simulink model "Tra_Prt"  (R2016b)
settings: configuration reference "CodeGenConfigSet" (kept outside this file)
values from neighbouring files (symbols this model uses):
  Tra_dtrqPTORmpP_Neg_C = Calibration.Parameter    [init_Tra_Prt.m]
  Tra_dtrqPTORmpP_Pos_C = Calibration.Parameter    [init_Tra_Prt.m]
  Tra_numGearGrpThres1_C = Calibration.Parameter    [init_Tra_Prt.m]
  Tra_numGearGrpThres2_C = Calibration.Parameter    [init_Tra_Prt.m]
  Tra_numGearGrpThres3_C = Calibration.Parameter    [init_Tra_Prt.m]
  Tra_numGearGrpThres4_C = Calibration.Parameter    [init_Tra_Prt.m]
  Tra_numGearGrpThres5_C = Calibration.Parameter    [init_Tra_Prt.m]
  Tra_swtPTOLim1KD_C = Calibration.Parameter    [init_Tra_Prt.m]
  Tra_trqInMax_C = Calibration.Parameter    [init_Tra_Prt.m]
  Tra_trqMaxGearGrp1_CUR = Calibration.Parameter    [init_Tra_Prt.m]
  Tra_trqMaxGearGrp1_CURX = Calibration.Parameter    [init_Tra_Prt.m]
  Tra_trqMaxGearGrp2_CUR = Calibration.Parameter    [init_Tra_Prt.m]
  Tra_trqMaxGearGrp2_CURX = Calibration.Parameter    [init_Tra_Prt.m]
  Tra_trqMaxGearGrp3_CUR = Calibration.Parameter    [init_Tra_Prt.m]
  Tra_trqMaxGearGrp3_CURX = Calibration.Parameter    [init_Tra_Prt.m]
  Tra_trqMaxGearGrp4_CUR = Calibration.Parameter    [init_Tra_Prt.m]
  Tra_trqMaxGearGrp4_CURX = Calibration.Parameter    [init_Tra_Prt.m]
  Tra_trqMaxGearGrp5_CUR = Calibration.Parameter    [init_Tra_Prt.m]
  Tra_trqMaxGearGrp5_CURX = Calibration.Parameter    [init_Tra_Prt.m]
  Tra_trqMaxGearGrp6_CUR = Calibration.Parameter    [init_Tra_Prt.m]
  Tra_trqMaxGearGrp6_CURX = Calibration.Parameter    [init_Tra_Prt.m]
  Tra_trqPTOLim1_CUR = Calibration.Parameter    [init_Tra_Prt.m]
  Tra_trqPTOLim1_CURX = Calibration.Parameter    [init_Tra_Prt.m]
  Tra_trqPTOLim2_CUR = Calibration.Parameter    [init_Tra_Prt.m]
  Tra_trqPTOLim2_CURX = Calibration.Parameter    [init_Tra_Prt.m]
  Tra_trqPTOLim3_CUR = Calibration.Parameter    [init_Tra_Prt.m]
  Tra_trqPTOLim3_CURX = Calibration.Parameter    [init_Tra_Prt.m]
  Tra_trqWESDemLim0_C = Calibration.Parameter    [init_Tra_Prt.m]
  Tra_trqWESDemLim1_C = Calibration.Parameter    [init_Tra_Prt.m]
  Tra_trqWESDemLim2_C = Calibration.Parameter    [init_Tra_Prt.m]
  Tra_trqWESDemLim3_C = Calibration.Parameter    [init_Tra_Prt.m]
undefined symbols (not defined in the file or in its folder): CEngDsT_tTransf_CURX, WESDem_State_conv
libraries: CXLib x1
settings Model: Creator=Colin  LastModifiedBy=wangrui
settings ConfigSetRef: SourceLocation=Base Workspace

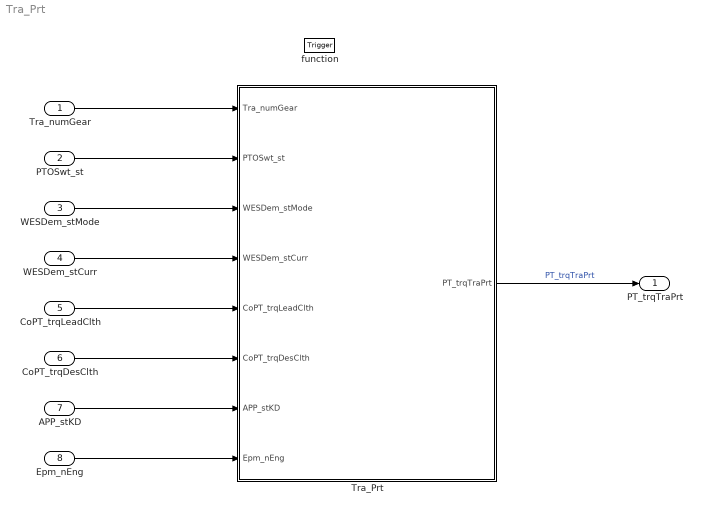
== system Tra_Prt ==
  Tra_numGear : Inport  Description=Current gear information  OutMin=-128  OutMax=127  OutDataTypeStr=Tra_num
  PTOSwt_st : Inport  Description=Power Take-off switch current state for a specific input voltage  Port=2  OutMin=0  OutMax=255  OutDataTypeStr=State_uint8
  WESDem_stMode : Inport  Description=Operating mode of the working engine speed demand  Port=3  OutMin=0  OutMax=255  OutDataTypeStr=State_uint8
  WESDem_stCurr : Inport  Description=Status of the working engine Speed Control  Port=4  OutDataTypeStr=Enum: WESDem_State_conv
  CoPT_trqLeadClth : Inport  Tag=Nm  Description=Lead torque demand at gearbox  Port=5  OutMin=-3000  OutMax=3000  OutDataTypeStr=Trq_Nm
  CoPT_trqDesClth : Inport  Tag=Nm  Description=Desired Clutch Torque  Port=6  OutMin=-3000  OutMax=3000  OutDataTypeStr=Trq_Nm
  APP_stKD : Inport  Description=State of accelerator pedal kick down  Port=7  OutMin=0  OutMax=1  OutDataTypeStr=boolean
  Epm_nEng : Inport  Tag=rpm  Description=Engine speed  Port=8  OutMin=0  OutMax=6000  OutDataTypeStr=EngSpeed_rpm
  function : TriggerPort  TriggerType=function-call  VariantControl=Variant
  Tra_Prt : Subsystem  RTWFcnName=Tra_Prt_Co  RTWFileName=Tra_Prt
      settings: RTWSystemCode=Nonreusable function  RTWFcnNameOpts=User specified  RTWFileNameOpts=User specified
  PT_trqTraPrt : Outport  Tag=Nm  Description=Maximum allowed inner torque  OutMin=-3000  OutMax=3000  OutDataTypeStr=Trq_Nm
  wires:
  Tra_Prt/1(PT_trqTraPrt) -> PT_trqTraPrt/1  "PT_trqTraPrt"
  Tra_numGear/1 -> Tra_Prt/1(Tra_numGear)
  PTOSwt_st/1 -> Tra_Prt/2(PTOSwt_st)
  WESDem_stMode/1 -> Tra_Prt/3(WESDem_stMode)
  WESDem_stCurr/1 -> Tra_Prt/4(WESDem_stCurr)
  CoPT_trqLeadClth/1 -> Tra_Prt/5(CoPT_trqLeadClth)
  APP_stKD/1 -> Tra_Prt/7(APP_stKD)
  CoPT_trqDesClth/1 -> Tra_Prt/6(CoPT_trqDesClth)
  Epm_nEng/1 -> Tra_Prt/8(Epm_nEng)

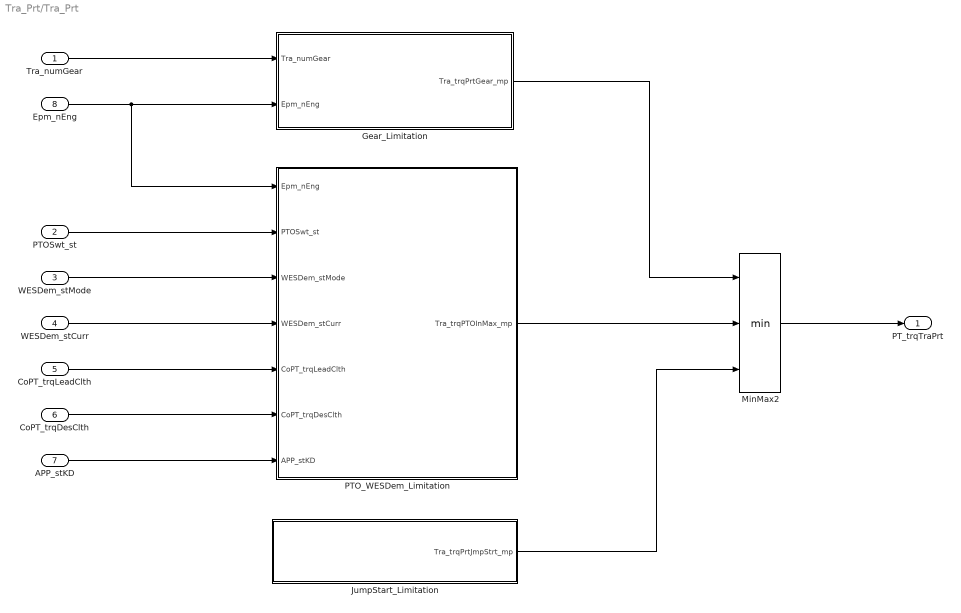
== system Tra_Prt/Tra_Prt ==
  Tra_numGear : Inport
  PTOSwt_st : Inport  Port=2
  WESDem_stMode : Inport  Port=3
  WESDem_stCurr : Inport  Port=4
  CoPT_trqLeadClth : Inport  Port=5
  CoPT_trqDesClth : Inport  Port=6
  APP_stKD : Inport  Port=7
  Epm_nEng : Inport  Port=8
  Gear_Limitation : Subsystem
  JumpStart_Limitation : Subsystem
  MinMax2 : MinMax  Inputs=3  InputSameDT=on
  PTO_WESDem_Limitation : Subsystem
  PT_trqTraPrt : Outport
  wires:
  Tra_numGear/1 -> Gear_Limitation/1(Tra_numGear)
  Gear_Limitation/1(Tra_trqPrtGear_mp) -> MinMax2/1
  MinMax2/1 -> PT_trqTraPrt/1
  APP_stKD/1 -> PTO_WESDem_Limitation/7(APP_stKD)
  CoPT_trqDesClth/1 -> PTO_WESDem_Limitation/6(CoPT_trqDesClth)
  PTO_WESDem_Limitation/1(Tra_trqPTOInMax_mp) -> MinMax2/2
  PTOSwt_st/1 -> PTO_WESDem_Limitation/2(PTOSwt_st)
  WESDem_stCurr/1 -> PTO_WESDem_Limitation/4(WESDem_stCurr)
  WESDem_stMode/1 -> PTO_WESDem_Limitation/3(WESDem_stMode)
  CoPT_trqLeadClth/1 -> PTO_WESDem_Limitation/5(CoPT_trqLeadClth)
  JumpStart_Limitation/1(Tra_trqPrtJmpStrt_mp) -> MinMax2/3
  Epm_nEng/1 -> PTO_WESDem_Limitation/1(Epm_nEng), Gear_Limitation/2(Epm_nEng)

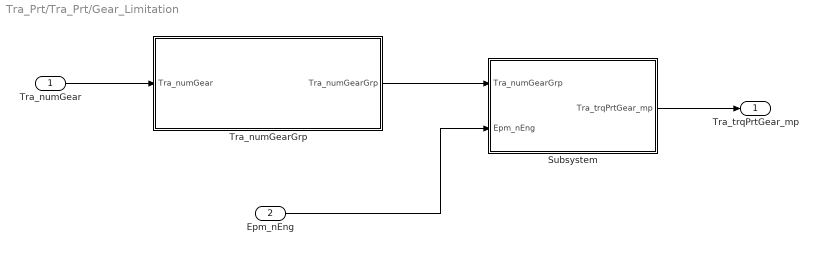
== system Tra_Prt/Tra_Prt/Gear_Limitation ==
  Tra_numGear : Inport
  Epm_nEng : Inport  Port=2
  Subsystem : Subsystem
  Tra_numGearGrp : Subsystem
  Tra_trqPrtGear_mp : Outport
  wires:
  Tra_numGear/1 -> Tra_numGearGrp/1(Tra_numGear)
  Tra_numGearGrp/1(Tra_numGearGrp) -> Subsystem/1(Tra_numGearGrp)
  Epm_nEng/1 -> Subsystem/2(Epm_nEng)
  Subsystem/1(Tra_trqPrtGear_mp) -> Tra_trqPrtGear_mp/1

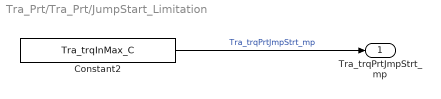
== system Tra_Prt/Tra_Prt/JumpStart_Limitation ==
  Constant2 : Constant  RequirementInfo={} %GIDa_d51cce05_4451_4a37_be15_ce81718d51d3  Value=Tra_trqInMax_C
  Tra_trqPrtJmpStrt_mp : Outport
  wires:
  Constant2/1 -> Tra_trqPrtJmpStrt_mp/1  "Tra_trqPrtJmpStrt_mp"

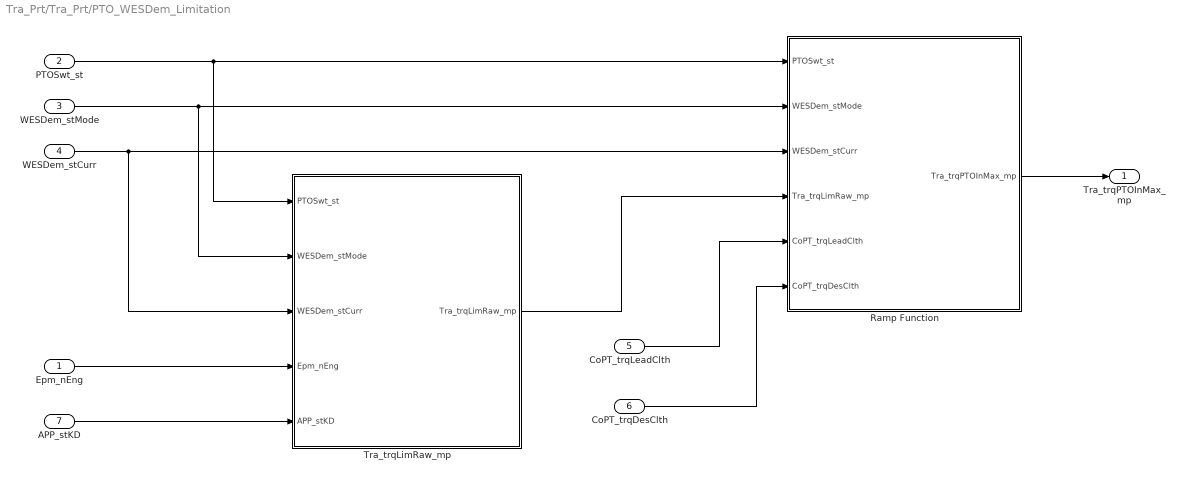
== system Tra_Prt/Tra_Prt/PTO_WESDem_Limitation ==
  Epm_nEng : Inport
  PTOSwt_st : Inport  Port=2
  WESDem_stMode : Inport  Port=3
  WESDem_stCurr : Inport  Port=4
  CoPT_trqLeadClth : Inport  Port=5
  CoPT_trqDesClth : Inport  Port=6
  APP_stKD : Inport  Port=7
  Ramp Function : Subsystem
  Tra_trqLimRaw_mp : Subsystem
  Tra_trqPTOInMax_mp : Outport
  wires:
  PTOSwt_st/1 -> Tra_trqLimRaw_mp/1(PTOSwt_st), Ramp Function/1(PTOSwt_st)
  WESDem_stMode/1 -> Tra_trqLimRaw_mp/2(WESDem_stMode), Ramp Function/2(WESDem_stMode)
  WESDem_stCurr/1 -> Tra_trqLimRaw_mp/3(WESDem_stCurr), Ramp Function/3(WESDem_stCurr)
  Ramp Function/1(Tra_trqPTOInMax_mp) -> Tra_trqPTOInMax_mp/1
  CoPT_trqLeadClth/1 -> Ramp Function/5(CoPT_trqLeadClth)
  CoPT_trqDesClth/1 -> Ramp Function/6(CoPT_trqDesClth)
  Epm_nEng/1 -> Tra_trqLimRaw_mp/4(Epm_nEng)
  APP_stKD/1 -> Tra_trqLimRaw_mp/5(APP_stKD)
  Tra_trqLimRaw_mp/1(Tra_trqLimRaw_mp) -> Ramp Function/4(Tra_trqLimRaw_mp)

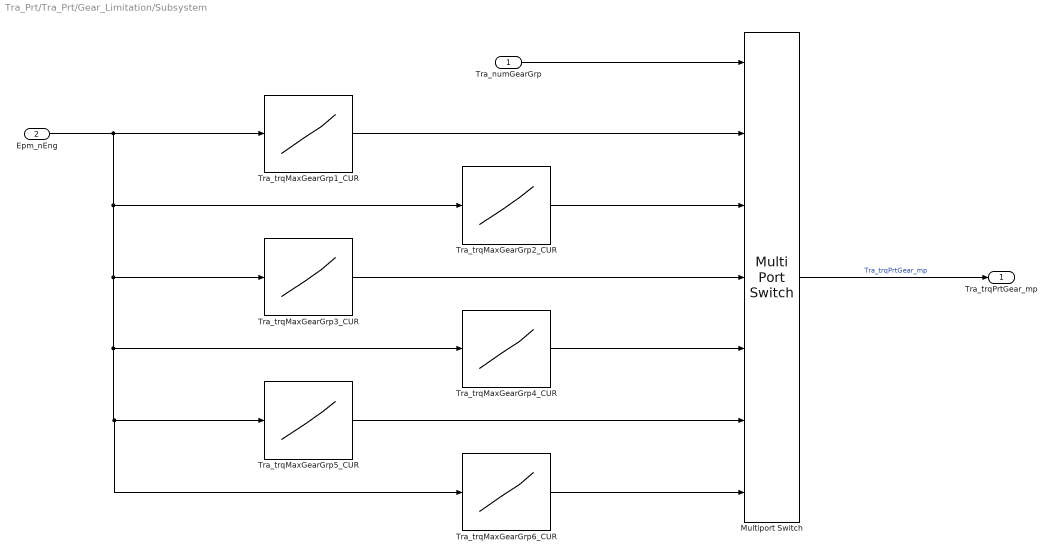
== system Tra_Prt/Tra_Prt/Gear_Limitation/Subsystem ==
  Tra_numGearGrp : Inport
  Epm_nEng : Inport  Port=2
  Multiport Switch : MultiPortSwitch  Inputs=6  InputSameDT=on
  Tra_trqMaxGearGrp1_CUR : Lookup_n-D  RequirementInfo={} %GIDa_9bf8303a_3058_4db5_a525_07331b8eeae7  DialogController=Simulink.DDGSource  NumberOfTableDimensions=1  BreakpointsForDimension1=Tra_trqMaxGearGrp1_CURX  BreakpointsForDimension2=CEngDsT_tTransf_CURX  IndexSearchMethod=Linear search  BeginIndexSearchUsingPreviousIndexResult=on  Table=Tra_trqMaxGearGrp1_CUR  ExtrapMethod=Clip  UseLastTableValue=on  InternalRulePriority=Speed  OutDataTypeStr=Inherit: Inherit via back propagation  SaturateOnIntegerOverflow=on
  Tra_trqMaxGearGrp2_CUR : Lookup_n-D  RequirementInfo={} %GIDa_3f32d6d9_4cb8_4f48_9c57_2c19b3164e61  DialogController=Simulink.DDGSource  NumberOfTableDimensions=1  BreakpointsForDimension1=Tra_trqMaxGearGrp2_CURX  BreakpointsForDimension2=CEngDsT_tTransf_CURX  IndexSearchMethod=Linear search  BeginIndexSearchUsingPreviousIndexResult=on  Table=Tra_trqMaxGearGrp2_CUR  ExtrapMethod=Clip  UseLastTableValue=on  InternalRulePriority=Speed  OutDataTypeStr=Inherit: Inherit via back propagation  SaturateOnIntegerOverflow=on
  Tra_trqMaxGearGrp3_CUR : Lookup_n-D  RequirementInfo={} %GIDa_1f71405c_5e82_4c6f_b5e1_f98a14c9db68  DialogController=Simulink.DDGSource  NumberOfTableDimensions=1  BreakpointsForDimension1=Tra_trqMaxGearGrp3_CURX  BreakpointsForDimension2=CEngDsT_tTransf_CURX  IndexSearchMethod=Linear search  BeginIndexSearchUsingPreviousIndexResult=on  Table=Tra_trqMaxGearGrp3_CUR  ExtrapMethod=Clip  UseLastTableValue=on  InternalRulePriority=Speed  OutDataTypeStr=Inherit: Inherit via back propagation  SaturateOnIntegerOverflow=on
  Tra_trqMaxGearGrp4_CUR : Lookup_n-D  RequirementInfo={} %GIDa_d67459b0_9d68_4b26_8ae3_ca0e9adf24a9  DialogController=Simulink.DDGSource  NumberOfTableDimensions=1  BreakpointsForDimension1=Tra_trqMaxGearGrp4_CURX  BreakpointsForDimension2=CEngDsT_tTransf_CURX  IndexSearchMethod=Linear search  BeginIndexSearchUsingPreviousIndexResult=on  Table=Tra_trqMaxGearGrp4_CUR  ExtrapMethod=Clip  UseLastTableValue=on  InternalRulePriority=Speed  OutDataTypeStr=Inherit: Inherit via back propagation  SaturateOnIntegerOverflow=on
  Tra_trqMaxGearGrp5_CUR : Lookup_n-D  RequirementInfo={} %GIDa_4c84db78_f469_4b3e_ba9a_5984f4299043  DialogController=Simulink.DDGSource  NumberOfTableDimensions=1  BreakpointsForDimension1=Tra_trqMaxGearGrp5_CURX  BreakpointsForDimension2=CEngDsT_tTransf_CURX  IndexSearchMethod=Linear search  BeginIndexSearchUsingPreviousIndexResult=on  Table=Tra_trqMaxGearGrp5_CUR  ExtrapMethod=Clip  UseLastTableValue=on  InternalRulePriority=Speed  OutDataTypeStr=Inherit: Inherit via back propagation  SaturateOnIntegerOverflow=on
  Tra_trqMaxGearGrp6_CUR : Lookup_n-D  RequirementInfo={} %GIDa_1b105f65_424f_42a0_97b6_462d21eb7e5b  DialogController=Simulink.DDGSource  NumberOfTableDimensions=1  BreakpointsForDimension1=Tra_trqMaxGearGrp6_CURX  BreakpointsForDimension2=CEngDsT_tTransf_CURX  IndexSearchMethod=Linear search  BeginIndexSearchUsingPreviousIndexResult=on  Table=Tra_trqMaxGearGrp6_CUR  ExtrapMethod=Clip  UseLastTableValue=on  InternalRulePriority=Speed  OutDataTypeStr=Inherit: Inherit via back propagation  SaturateOnIntegerOverflow=on
  Tra_trqPrtGear_mp : Outport
  wires:
  Tra_numGearGrp/1 -> Multiport Switch/1
  Multiport Switch/1 -> Tra_trqPrtGear_mp/1  "Tra_trqPrtGear_mp"
  Tra_trqMaxGearGrp3_CUR/1 -> Multiport Switch/4
  Tra_trqMaxGearGrp4_CUR/1 -> Multiport Switch/5
  Epm_nEng/1 -> Tra_trqMaxGearGrp1_CUR/1, Tra_trqMaxGearGrp2_CUR/1, Tra_trqMaxGearGrp5_CUR/1, Tra_trqMaxGearGrp6_CUR/1, Tra_trqMaxGearGrp4_CUR/1, Tra_trqMaxGearGrp3_CUR/1
  Tra_trqMaxGearGrp6_CUR/1 -> Multiport Switch/7
  Tra_trqMaxGearGrp1_CUR/1 -> Multiport Switch/2
  Tra_trqMaxGearGrp5_CUR/1 -> Multiport Switch/6
  Tra_trqMaxGearGrp2_CUR/1 -> Multiport Switch/3

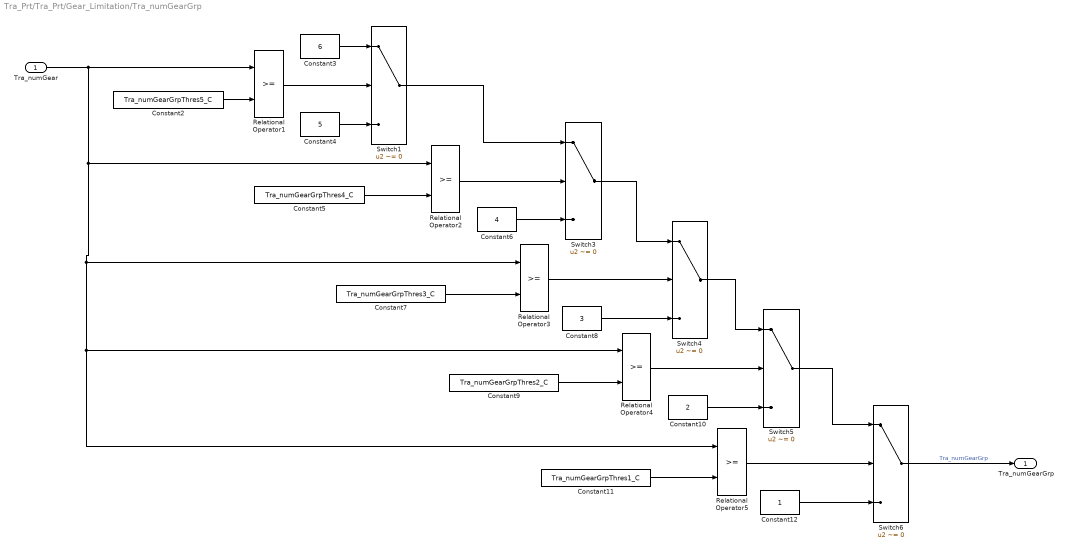
== system Tra_Prt/Tra_Prt/Gear_Limitation/Tra_numGearGrp ==
  Tra_numGear : Inport
  Constant10 : Constant  RequirementInfo={} %GIDa_cc2dd223_55c8_4d93_b3af_451ceaa6fd87  Value=2  OutDataTypeStr=Inherit: Inherit via back propagation
  Constant11 : Constant  RequirementInfo={} %GIDa_e35aa74d_c22f_4faf_ad9e_62e3164d3ca4  Value=Tra_numGearGrpThres1_C
  Constant12 : Constant  RequirementInfo={} %GIDa_f1b5e830_831e_49bb_af2f_76cdb3eefdd3  OutDataTypeStr=Inherit: Inherit via back propagation
  Constant2 : Constant  RequirementInfo={} %GIDa_3dc0d41d_75cf_443b_8b3e_59d12e38bafb  Value=Tra_numGearGrpThres5_C
  Constant3 : Constant  RequirementInfo={} %GIDa_e56e3a48_16bc_4fb2_9a60_cf299b0ddc0c  Value=6  OutDataTypeStr=Inherit: Inherit via back propagation
  Constant4 : Constant  RequirementInfo={} %GIDa_a586fa19_184d_42cb_966b_ca70260552d9  Value=5  OutDataTypeStr=Inherit: Inherit via back propagation
  Constant5 : Constant  RequirementInfo={} %GIDa_b9c0ff5b_d8f4_46d0_9cf8_05ffc9512e3e  Value=Tra_numGearGrpThres4_C
  Constant6 : Constant  RequirementInfo={} %GIDa_931eede9_2f33_482c_88fc_d1f4a7460dde  Value=4  OutDataTypeStr=Inherit: Inherit via back propagation
  Constant7 : Constant  RequirementInfo={} %GIDa_8d38ea8f_739b_430c_9a0e_9b66a82047ad  Value=Tra_numGearGrpThres3_C
  Constant8 : Constant  RequirementInfo={} %GIDa_3631fbf9_fa7a_45cb_b172_853493309744  Value=3  OutDataTypeStr=Inherit: Inherit via back propagation
  Constant9 : Constant  RequirementInfo={} %GIDa_7790a0c3_045c_47a2_950a_5d283818d59e  Value=Tra_numGearGrpThres2_C
  Relational Operator{1..5} (5 alike) : RelationalOperator  OutDataTypeStr=boolean  RndMeth=Simplest  InputSameDT=on
  Switch{1,3..6} (5 alike) : Switch  Criteria=u2 ~= 0  InputSameDT=on
  Tra_numGearGrp : Outport
  wires:
  Constant8/1 -> Switch4/3
  Constant10/1 -> Switch5/3
  Relational Operator5/1 -> Switch6/2
  Constant11/1 -> Relational Operator5/2
  Switch5/1 -> Switch6/1
  Constant5/1 -> Relational Operator2/2
  Tra_numGear/1 -> Relational Operator1/1, Relational Operator5/1, Relational Operator4/1, Relational Operator3/1, Relational Operator2/1
  Switch1/1 -> Switch3/1
  Switch3/1 -> Switch4/1
  Constant7/1 -> Relational Operator3/2
  Constant9/1 -> Relational Operator4/2
  Constant4/1 -> Switch1/3
  Relational Operator3/1 -> Switch4/2
  Relational Operator1/1 -> Switch1/2
  Constant6/1 -> Switch3/3
  Switch6/1 -> Tra_numGearGrp/1  "Tra_numGearGrp"
  Switch4/1 -> Switch5/1
  Relational Operator4/1 -> Switch5/2
  Constant12/1 -> Switch6/3
  Constant3/1 -> Switch1/1
  Relational Operator2/1 -> Switch3/2
  Constant2/1 -> Relational Operator1/2

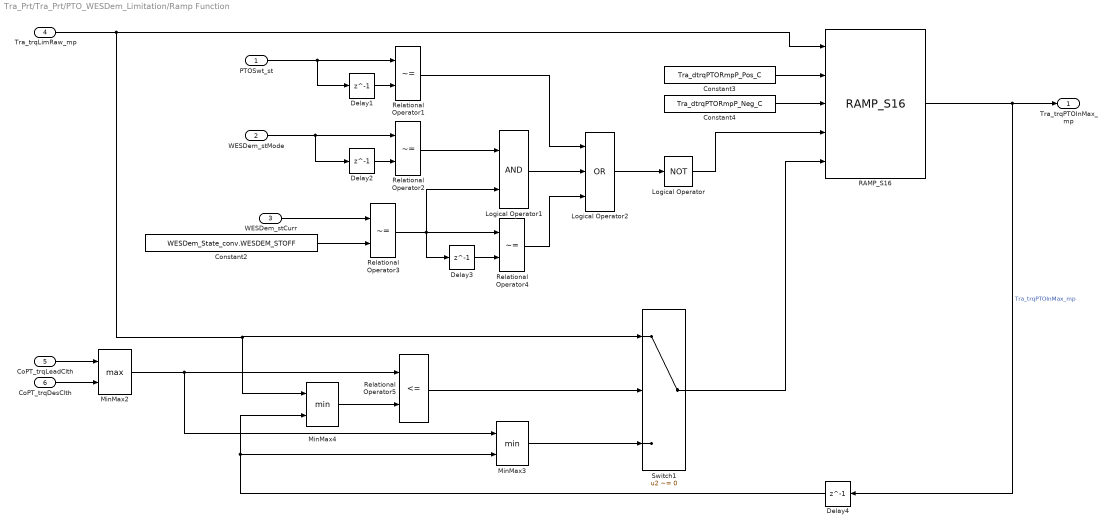
== system Tra_Prt/Tra_Prt/PTO_WESDem_Limitation/Ramp Function ==
  PTOSwt_st : Inport
  WESDem_stMode : Inport  Port=2
  WESDem_stCurr : Inport  Port=3
  Tra_trqLimRaw_mp : Inport  Port=4
  CoPT_trqLeadClth : Inport  Port=5
  CoPT_trqDesClth : Inport  Port=6
  Constant2 : Constant  RequirementInfo={} %GIDa_466aa6c1_d4cb_4c5d_8671_5e76f2249d25  Value=WESDem_State_conv.WESDEM_STOFF
  Constant3 : Constant  RequirementInfo={} %GIDa_db27a465_98ec_4314_b6ef_f20a25fea807  Value=Tra_dtrqPTORmpP_Pos_C
  Constant4 : Constant  RequirementInfo={} %GIDa_4651a11a_0cc9_4270_9106_49cbf50b5a07  Value=Tra_dtrqPTORmpP_Neg_C
  Delay{1..4} (4 alike) : Delay  DelayLength=1  InitialCondition=0
  Logical Operator : Logic  Operator=NOT  AllPortsSameDT=off  OutDataTypeStr=boolean
  Logical Operator1 : Logic  AllPortsSameDT=off  OutDataTypeStr=boolean
  Logical Operator2 : Logic  Operator=OR  Inputs=3  OutDataTypeStr=boolean
  MinMax2 : MinMax  Function=max  Inputs=2  InputSameDT=on
  MinMax3 : MinMax  Inputs=2  InputSameDT=on
  MinMax4 : MinMax  Inputs=2  InputSameDT=on
  RAMP_S16 : CXLib/RAMP_S16
  Relational Operator{1..4} (4 alike) : RelationalOperator  Operator=~=  OutDataTypeStr=boolean  RndMeth=Simplest  InputSameDT=on
  Relational Operator5 : RelationalOperator  Operator=<=  OutDataTypeStr=boolean  RndMeth=Simplest  InputSameDT=on
  Switch1 : Switch  Criteria=u2 ~= 0  InputSameDT=on
  Tra_trqPTOInMax_mp : Outport
  wires:
  Relational Operator5/1 -> Switch1/2
  Relational Operator3/1 -> Logical Operator1/2, Relational Operator4/1, Delay3/1
  Logical Operator1/1 -> Logical Operator2/2
  Delay3/1 -> Relational Operator4/2
  Relational Operator2/1 -> Logical Operator1/1
  Relational Operator4/1 -> Logical Operator2/3
  Relational Operator1/1 -> Logical Operator2/1
  Delay2/1 -> Relational Operator2/2
  Delay1/1 -> Relational Operator1/2
  WESDem_stMode/1 -> Relational Operator2/1, Delay2/1
  WESDem_stCurr/1 -> Relational Operator3/1
  Constant2/1 -> Relational Operator3/2
  PTOSwt_st/1 -> Relational Operator1/1, Delay1/1
  RAMP_S16/1 -> Tra_trqPTOInMax_mp/1, Delay4/1  "Tra_trqPTOInMax_mp"
  Constant3/1 -> RAMP_S16/2
  Constant4/1 -> RAMP_S16/3
  CoPT_trqDesClth/1 -> MinMax2/2
  MinMax4/1 -> Relational Operator5/2
  Tra_trqLimRaw_mp/1 -> RAMP_S16/1, Switch1/1, MinMax4/1
  Switch1/1 -> RAMP_S16/5
  Delay4/1 -> MinMax3/2, MinMax4/2
  MinMax3/1 -> Switch1/3
  MinMax2/1 -> MinMax3/1, Relational Operator5/1
  CoPT_trqLeadClth/1 -> MinMax2/1
  Logical Operator2/1 -> Logical Operator/1
  Logical Operator/1 -> RAMP_S16/4

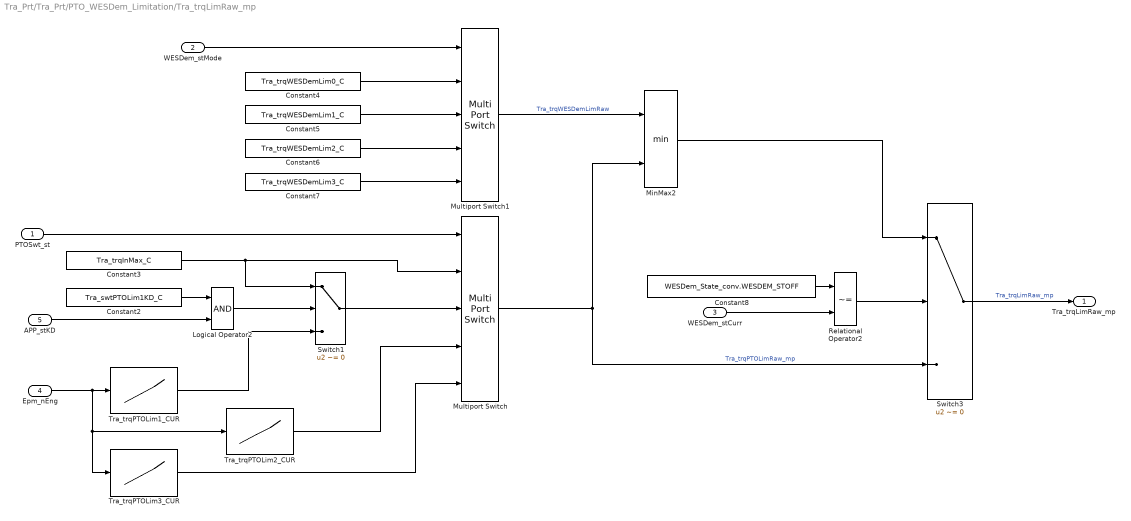
== system Tra_Prt/Tra_Prt/PTO_WESDem_Limitation/Tra_trqLimRaw_mp ==
  PTOSwt_st : Inport
  WESDem_stMode : Inport  Port=2
  WESDem_stCurr : Inport  Port=3
  Epm_nEng : Inport  Port=4
  APP_stKD : Inport  Port=5
  Constant2 : Constant  RequirementInfo={} %GIDa_3f12df52_063e_4b6b_83ab_e7f38802d6f3  Value=Tra_swtPTOLim1KD_C
  Constant3 : Constant  RequirementInfo={} %GIDa_c8f050d6_2e98_4ef5_be6e_79fb3d4a7b6f  Value=Tra_trqInMax_C
  Constant4 : Constant  RequirementInfo={} %GIDa_c56981e5_bb1f_4d21_91c2_b22ebc23756d  Value=Tra_trqWESDemLim0_C
  Constant5 : Constant  RequirementInfo={} %GIDa_c86881d6_7d68_4884_a96f_37f337ecea53  Value=Tra_trqWESDemLim1_C
  Constant6 : Constant  RequirementInfo={} %GIDa_d963e073_852e_4195_bb58_4ba7e0c59777  Value=Tra_trqWESDemLim2_C
  Constant7 : Constant  RequirementInfo={} %GIDa_b7ca61a4_d579_409a_88b6_94f397f03f6d  Value=Tra_trqWESDemLim3_C
  Constant8 : Constant  RequirementInfo={} %GIDa_c0306a82_42bc_47e8_a062_55d6454bf448  Value=WESDem_State_conv.WESDEM_STOFF
  Logical Operator2 : Logic  OutDataTypeStr=boolean
  MinMax2 : MinMax  Inputs=2  InputSameDT=on
  Multiport Switch : MultiPortSwitch  DataPortOrder=Specify indices  Inputs=4  DataPortIndices={0,1,2,3}
  Multiport Switch1 : MultiPortSwitch  DataPortOrder=Specify indices  Inputs=4  DataPortIndices={0,1,2,3}
  Relational Operator2 : RelationalOperator  Operator=~=  OutDataTypeStr=boolean  RndMeth=Simplest  InputSameDT=on
  Switch1 : Switch  Criteria=u2 ~= 0  InputSameDT=on
  Switch3 : Switch  Criteria=u2 ~= 0  InputSameDT=on
  Tra_trqPTOLim1_CUR : Lookup_n-D  RequirementInfo={} %GIDa_6194a397_485f_41d0_9768_b516be8cda6f  DialogController=Simulink.DDGSource  NumberOfTableDimensions=1  BreakpointsForDimension1=Tra_trqPTOLim1_CURX  BreakpointsForDimension2=CEngDsT_tTransf_CURX  IndexSearchMethod=Linear search  BeginIndexSearchUsingPreviousIndexResult=on  Table=Tra_trqPTOLim1_CUR  ExtrapMethod=Clip  UseLastTableValue=on  InternalRulePriority=Speed  OutDataTypeStr=Inherit: Inherit via back propagation  SaturateOnIntegerOverflow=on
  Tra_trqPTOLim2_CUR : Lookup_n-D  RequirementInfo={} %GIDa_e4df92cf_0072_4bb0_b948_3e03f5a56770  DialogController=Simulink.DDGSource  NumberOfTableDimensions=1  BreakpointsForDimension1=Tra_trqPTOLim2_CURX  BreakpointsForDimension2=CEngDsT_tTransf_CURX  IndexSearchMethod=Linear search  BeginIndexSearchUsingPreviousIndexResult=on  Table=Tra_trqPTOLim2_CUR  ExtrapMethod=Clip  UseLastTableValue=on  InternalRulePriority=Speed  OutDataTypeStr=Inherit: Inherit via back propagation  SaturateOnIntegerOverflow=on
  Tra_trqPTOLim3_CUR : Lookup_n-D  RequirementInfo={} %GIDa_60ae4370_cc59_41d5_93d4_1ec26251eec2  DialogController=Simulink.DDGSource  NumberOfTableDimensions=1  BreakpointsForDimension1=Tra_trqPTOLim3_CURX  BreakpointsForDimension2=CEngDsT_tTransf_CURX  IndexSearchMethod=Linear search  BeginIndexSearchUsingPreviousIndexResult=on  Table=Tra_trqPTOLim3_CUR  ExtrapMethod=Clip  UseLastTableValue=on  InternalRulePriority=Speed  OutDataTypeStr=Inherit: Inherit via back propagation  SaturateOnIntegerOverflow=on
  Tra_trqLimRaw_mp : Outport
  wires:
  Constant2/1 -> Logical Operator2/1
  Constant4/1 -> Multiport Switch1/2
  Constant7/1 -> Multiport Switch1/5
  Tra_trqPTOLim2_CUR/1 -> Multiport Switch/4
  Constant8/1 -> Relational Operator2/1
  WESDem_stCurr/1 -> Relational Operator2/2
  Logical Operator2/1 -> Switch1/2
  Switch1/1 -> Multiport Switch/3
  Multiport Switch/1 -> MinMax2/2, Switch3/3  "Tra_trqPTOLimRaw_mp"
  Constant3/1 -> Multiport Switch/2, Switch1/1
  PTOSwt_st/1 -> Multiport Switch/1
  Tra_trqPTOLim3_CUR/1 -> Multiport Switch/5
  MinMax2/1 -> Switch3/1
  Relational Operator2/1 -> Switch3/2
  Constant5/1 -> Multiport Switch1/3
  Constant6/1 -> Multiport Switch1/4
  WESDem_stMode/1 -> Multiport Switch1/1
  Epm_nEng/1 -> Tra_trqPTOLim3_CUR/1, Tra_trqPTOLim2_CUR/1, Tra_trqPTOLim1_CUR/1
  Tra_trqPTOLim1_CUR/1 -> Switch1/3
  Switch3/1 -> Tra_trqLimRaw_mp/1  "Tra_trqLimRaw_mp"
  APP_stKD/1 -> Logical Operator2/2
  Multiport Switch1/1 -> MinMax2/1  "Tra_trqWESDemLimRaw"
